simulink model "slModelRDBRx"  (R2015a)
settings: Solver=ode3  StartTime=0.0  StopTime=1000000  FixedStep=1  RelTol=1e-3
libraries: simulink x2
settings Model: Creator=holger  LastModifiedBy=holger

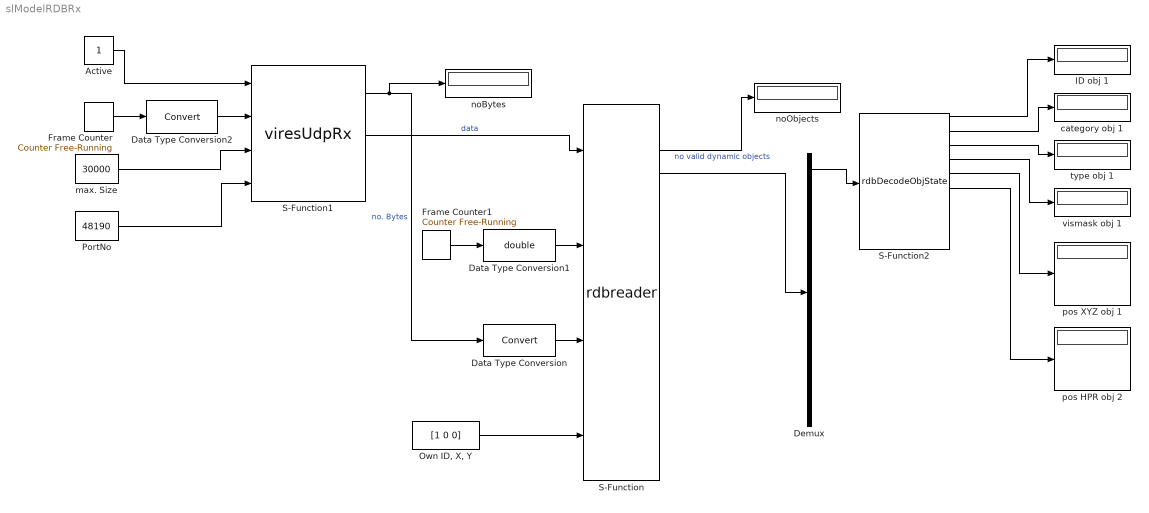
== system slModelRDBRx ==
  Active : Constant  OutDataTypeStr=uint32
  Data Type Conversion : DataTypeConversion
  Data Type Conversion1 : DataTypeConversion  OutDataTypeStr=double
  Data Type Conversion2 : DataTypeConversion
  Demux : Demux  Outputs=20
  Frame Counter : simulink/Sources/Counter Free-Running  NumBits=16  tsamp=-1
  Frame Counter1 : simulink/Sources/Counter Free-Running  NumBits=16  tsamp=-1
  ID obj 1 : Display
  "Own ID, X, Y" : Constant  Value=[1 0 0]  OutDataTypeStr=double
  PortNo : Constant  Value=48190  OutDataTypeStr=uint32
  S-Function : S-Function  FunctionName=rdbreader
  S-Function1 : S-Function  FunctionName=viresUdpRx
  S-Function2 : S-Function  FunctionName=rdbDecodeObjState
  category obj 1 : Display
  max. Size : Constant  Value=30000  OutDataTypeStr=uint32
  noBytes : Display
  noObjects : Display
  pos HPR obj 2 : Display
  pos XYZ obj 1 : Display
  type obj 1 : Display
  vismask obj 1 : Display
  wires:
  S-Function/2 -> noObjects/1  "no valid dynamic objects"
  S-Function1/2 -> S-Function/1  "data"
  S-Function1/1 -> noBytes/1, Data Type Conversion/1  "no. Bytes"
  Active/1 -> S-Function1/1
  PortNo/1 -> S-Function1/4
  "Own ID, X, Y"/1 -> S-Function/4
  Data Type Conversion/1 -> S-Function/3
  Data Type Conversion1/1 -> S-Function/2
  Frame Counter1/1 -> Data Type Conversion1/1
  Data Type Conversion2/1 -> S-Function1/2
  Frame Counter/1 -> Data Type Conversion2/1
  max. Size/1 -> S-Function1/3
  S-Function/3 -> Demux/1
  S-Function2/2 -> category obj 1/1
  S-Function2/1 -> ID obj 1/1
  S-Function2/3 -> type obj 1/1
  S-Function2/4 -> vismask obj 1/1
  S-Function2/5 -> pos XYZ obj 1/1
  S-Function2/6 -> pos HPR obj 2/1
  Demux/2 -> S-Function2/1
